simulink model "sim_prbs"  (R2015a)
settings: Solver=ode45  StartTime=0.0  StopTime=300  RelTol=1e-3
libraries: simulink_extras x1
settings Model: Creator=n221  LastModifiedBy=n221

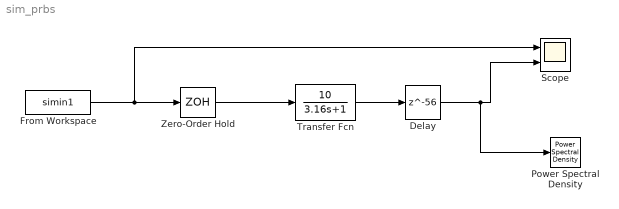
== system sim_prbs ==
  Delay : Delay  DelayLength=56  SampleTime=0.01
  From Workspace : FromWorkspace  VariableName=simin1  SampleTime=0.01
  Power Spectral Density : simulink_extras/Additional Sinks/Power Spectral Density  npts=128  fftpts=512  HowOften=64  sampleT=0.1
  Scope : Scope  NumInputPorts=2
      settings: YMin=-5~-5  YMax=5~5  SaveName=datos
  Transfer Fcn : TransferFcn  Numerator=[10]  Denominator=[3.16 1]
  Zero-Order Hold : ZeroOrderHold  SampleTime=0.01
  wires:
  From Workspace/1 -> Scope/1, Zero-Order Hold/1
  Zero-Order Hold/1 -> Transfer Fcn/1
  Transfer Fcn/1 -> Delay/1
  Delay/1 -> Power Spectral Density/1, Scope/2
